simulink model "eml_2nd_order_filter"  (Simulink 7.7)
settings: Solver=FixedStepDiscrete  StartTime=0.0  StopTime=1  RelTol=1e-3
values from neighbouring files (symbols this model uses):
  den = [1                  -1.4542435862515900  0.5740619150839550]    [fi_instrumentation_fixed_point_filter_demo.m]
  num = [0.0299545822080925  0.0599091644161849  0.0299545822080925]    [fi_instrumentation_fixed_point_filter_demo.m]
libraries: simulink x1
settings Model: Creator=tbryan  LastModifiedBy=kbackhou  ExtModeAutoUpdateStatusClock=off
settings OptimizationCC: InitFltsAndDblsToZero=on
settings DebuggingCC: SaveWithParameterizedLinksMsg=none  SignalResolutionControl=TryResolveAllWithWarning  MultiTaskDSMMsg=warning  MultiTaskCondExecSysMsg=none  SigSpecEnsureSampleTimeMsg=none  IntegerOverflowMsg=none  Int32ToFloatConvMsg=none  ParameterOverflowMsg=none  ParameterPrecisionLossMsg=none  StrictBusMsg=Warning
settings SFSimCC: SimParseCustomCode=off
settings RTWCC: IncludeERTFirstTime=on
settings GRTTargetCC: TargetFcnLib=ansi_tfl_tmw.mat

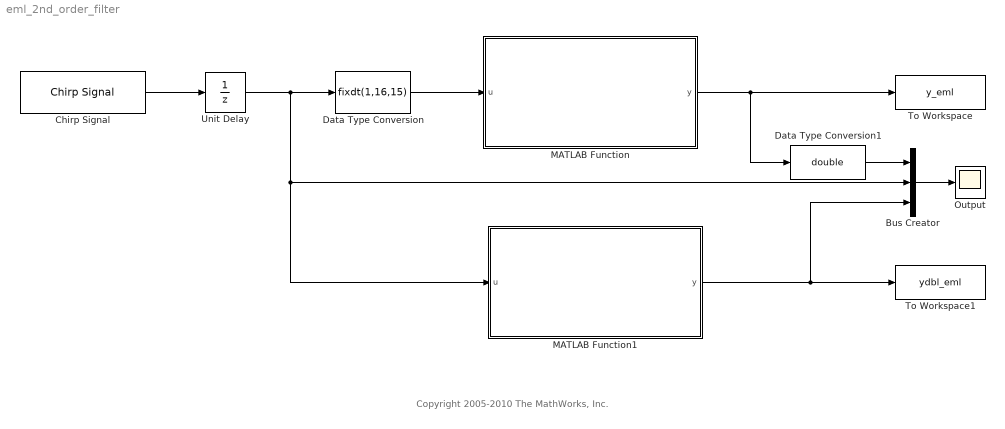
== system eml_2nd_order_filter ==
  note: Copyright 2005-2010 The MathWorks, Inc.
  Bus Creator : BusCreator  Inputs=3
  Chirp Signal : simulink/Sources/Chirp Signal  SystemSampleTime=-1  f1=0  T=1  f2=128
  Data Type Conversion : DataTypeConversion  OutDataTypeStr=fixdt(1,16,15)  RndMeth=Nearest  SaturateOnIntegerOverflow=on
  Data Type Conversion1 : DataTypeConversion  OutDataTypeStr=double  RndMeth=Nearest  SaturateOnIntegerOverflow=on
  MATLAB Function : Stateflow chart  TreatAsAtomicUnit=on
  MATLAB Function1 : Stateflow chart  TreatAsAtomicUnit=on
  Output : Scope
      settings: TimeRange=1
  To Workspace : ToWorkspace  VariableName=y_eml  SampleTime=-1  SaveFormat=Array
  To Workspace1 : ToWorkspace  VariableName=ydbl_eml  SampleTime=-1  SaveFormat=Array
  Unit Delay : UnitDelay  SampleTime=1/256
  wires:
  Chirp Signal/1 -> Unit Delay/1
  Data Type Conversion/1 -> MATLAB Function/1(u)
  Bus Creator/1 -> Output/1
  MATLAB Function/1(y) -> To Workspace/1, Data Type Conversion1/1
  Unit Delay/1 -> Data Type Conversion/1, Bus Creator/2, MATLAB Function1/1(u)
  MATLAB Function1/1(y) -> To Workspace1/1, Bus Creator/3
  Data Type Conversion1/1 -> Bus Creator/1

== matlab function MATLAB Function1 ==
  settings: fimath=fimath;
  data: num parameter double; den parameter double; u input double; y output double
function y = fi_2nd_order_filter(num, den, u)
%#codegen

y = fieml_2nd_order_filter(num, den, u);

== matlab function MATLAB Function ==
  settings: fimath=fimath;
  data: num parameter double; den parameter double; u input double; y output double
function y = fi_2nd_order_filter(num, den, u)
%#codegen

y = fieml_2nd_order_filter(num,den,u);
